simulink model "magnetorquer"  (R2019a)
settings: Solver=ode5  StartTime=0.0  StopTime=10.0  RelTol=1e-3
undefined symbols (not defined in the file or in its folder): sat
libraries: sharedutil x4, simulink x3, vrlib x1
settings Model: Creator=Florian  LastModifiedBy=Florian

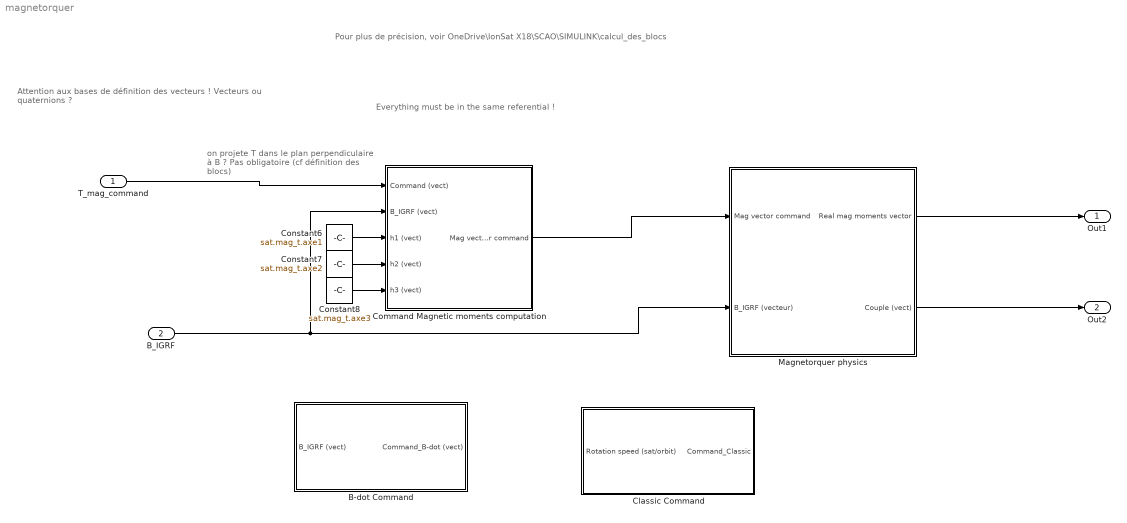
== system magnetorquer ==
  note: Attention aux bases de définition des vecteurs !
      |
      | Vecteurs ou quaternions ?
  note: on projete T dans
      | le plan perpendiculaire à B ?
      | Pas obligatoire (cf définition des blocs)
  note: Everything must be in the same referential !
  note: Pour plus de précision, voir OneDrive\IonSat X18\SCAO\SIMULINK\calcul_des_blocs
  T_mag_command : Inport
  B_IGRF : Inport  Port=2
  B-dot Command : Subsystem
  Classic Command : Subsystem
  Command Magnetic moments computation : Subsystem
  Constant6 : Constant  Value=sat.mag_t.axe1
  Constant7 : Constant  Value=sat.mag_t.axe2
  Constant8 : Constant  Value=sat.mag_t.axe3
  Magnetorquer physics : Subsystem
  Out1 : Outport
  Out2 : Outport  Port=2
  wires:
  Magnetorquer physics/1(Real mag moments vector) -> Out1/1
  Magnetorquer physics/2(Couple (vect)) -> Out2/1
  B_IGRF/1 -> Magnetorquer physics/2(B_IGRF (vecteur)), Command Magnetic moments computation/2(B_IGRF (vect))
  T_mag_command/1 -> Command Magnetic moments computation/1(Command (vect))
  Constant6/1 -> Command Magnetic moments computation/3(h1 (vect))
  Constant7/1 -> Command Magnetic moments computation/4(h2 (vect))
  Constant8/1 -> Command Magnetic moments computation/5(h3 (vect))
  Command Magnetic moments computation/1(Mag vector command) -> Magnetorquer physics/1(Mag vector command)

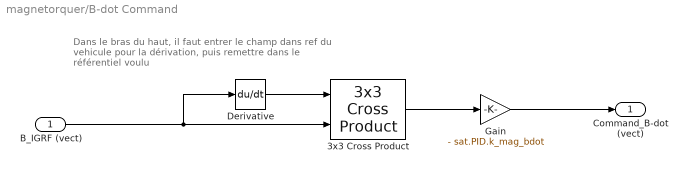
== system magnetorquer/B-dot Command ==
  note: Dans le bras du haut, il faut entrer le champ
      | dans ref du vehicule pour la dérivation, puis remettre
      | dans le référentiel voulu
  B_IGRF (vect) : Inport
  3x3 Cross Product : sharedutil/3x3 Cross Product  aMode=aMode
      settings: SourceProductBaseCode=AE
  Derivative : Derivative
  Gain : Gain  Gain=- sat.PID.k_mag_bdot
  Command_B-dot (vect) : Outport  VectorParamsAs1DForOutWhenUnconnected=off
  wires:
  Derivative/1 -> 3x3 Cross Product/1
  Gain/1 -> Command_B-dot (vect)/1
  B_IGRF (vect)/1 -> Derivative/1, 3x3 Cross Product/2
  3x3 Cross Product/1 -> Gain/1

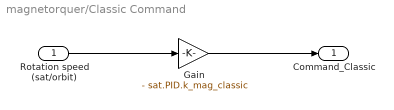
== system magnetorquer/Classic Command ==
  Rotation speed (sat/orbit) : Inport
  Gain : Gain  Gain=- sat.PID.k_mag_classic
  Command_Classic : Outport  VectorParamsAs1DForOutWhenUnconnected=off
  wires:
  Rotation speed (sat/orbit)/1 -> Gain/1
  Gain/1 -> Command_Classic/1

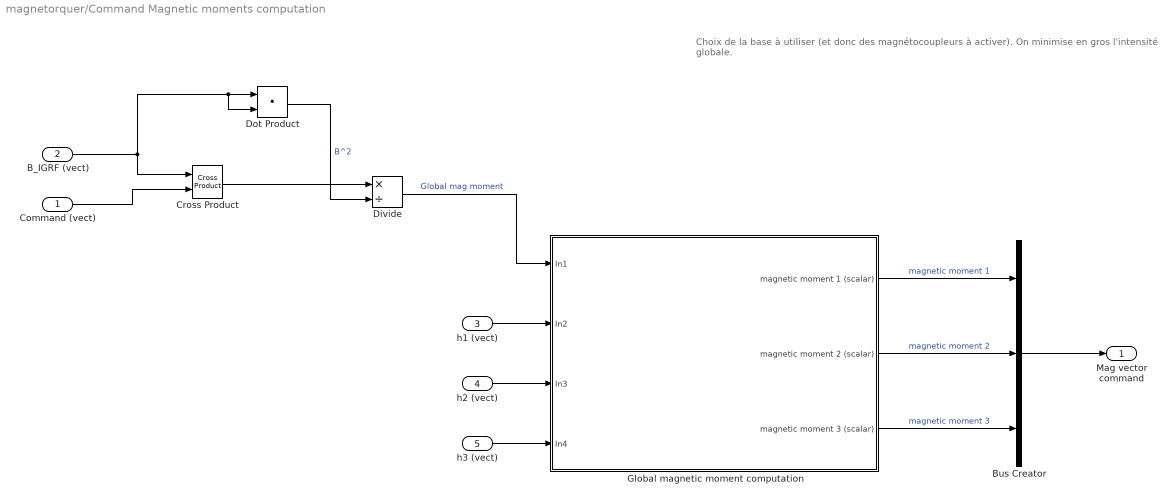
== system magnetorquer/Command Magnetic moments computation ==
  note: Choix de la base à utiliser (et donc des magnétocoupleurs à activer). On minimise en gros l'intensité globale.
  Command (vect) : Inport
  B_IGRF (vect) : Inport  Port=2
  h1 (vect) : Inport  Port=3
  h2 (vect) : Inport  Port=4
  h3 (vect) : Inport  Port=5
  Bus Creator : BusCreator  Inputs=3
  Cross Product : vrlib/Utilities/Cross Product
      settings: SourceProductName=Simulink
  Divide : Product  Inputs=*/
  Dot Product : DotProduct  InputSameDT=on  OutDataTypeStr=Inherit: Inherit via internal rule
  Global magnetic moment computation : Subsystem
  Mag vector command : Outport  VectorParamsAs1DForOutWhenUnconnected=off
  wires:
  B_IGRF (vect)/1 -> Dot Product/2, Dot Product/1, Cross Product/1
  Command (vect)/1 -> Cross Product/2
  Dot Product/1 -> Divide/2  "B^2"
  Cross Product/1 -> Divide/1
  Divide/1 -> Global magnetic moment computation/1(In1)  "Global mag moment"
  h1 (vect)/1 -> Global magnetic moment computation/2(In2)
  h2 (vect)/1 -> Global magnetic moment computation/3(In3)
  h3 (vect)/1 -> Global magnetic moment computation/4(In4)
  Global magnetic moment computation/2(magnetic moment 2 (scalar)) -> Bus Creator/2  "magnetic moment 2"
  Global magnetic moment computation/3(magnetic moment 3 (scalar)) -> Bus Creator/3  "magnetic moment 3"
  Global magnetic moment computation/1(magnetic moment 1 (scalar)) -> Bus Creator/1  "magnetic moment 1"
  Bus Creator/1 -> Mag vector command/1

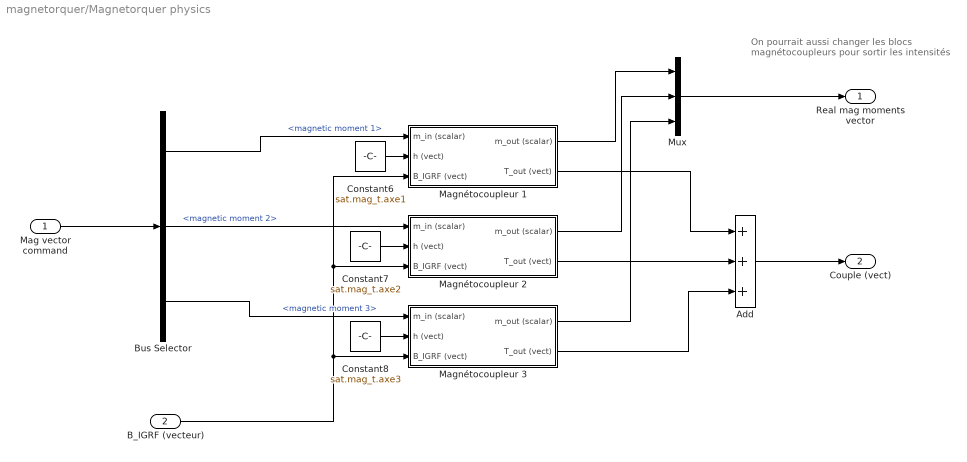
== system magnetorquer/Magnetorquer physics ==
  note: On pourrait aussi changer les blocs
      | magnétocoupleurs pour sortir les intensités
  Mag vector command : Inport
  B_IGRF (vecteur) : Inport  Port=2
  Add : Sum  Inputs=+++
  Bus Selector : BusSelector  OutputSignals=magnetic moment 1,magnetic moment 2,magnetic moment 3
  Constant6 : Constant  Value=sat.mag_t.axe1
  Constant7 : Constant  Value=sat.mag_t.axe2
  Constant8 : Constant  Value=sat.mag_t.axe3
  Magnétocoupleur 1 : Subsystem
  Magnétocoupleur 2 : Subsystem
  Magnétocoupleur 3 : Subsystem
  Mux : Mux  Inputs=3
  Real mag moments vector : Outport  VectorParamsAs1DForOutWhenUnconnected=off
  Couple (vect) : Outport  Port=2  VectorParamsAs1DForOutWhenUnconnected=off
  wires:
  Constant6/1 -> Magnétocoupleur 1/2(h (vect))
  B_IGRF (vecteur)/1 -> Magnétocoupleur 1/3(B_IGRF (vect)), Magnétocoupleur 2/3(B_IGRF (vect)), Magnétocoupleur 3/3(B_IGRF (vect))
  Constant7/1 -> Magnétocoupleur 2/2(h (vect))
  Magnétocoupleur 2/1(m_out (scalar)) -> Mux/2
  Add/1 -> Couple (vect)/1
  Magnétocoupleur 1/2(T_out (vect)) -> Add/1
  Magnétocoupleur 2/2(T_out (vect)) -> Add/2
  Magnétocoupleur 3/2(T_out (vect)) -> Add/3
  Mux/1 -> Real mag moments vector/1
  Magnétocoupleur 1/1(m_out (scalar)) -> Mux/1
  Magnétocoupleur 3/1(m_out (scalar)) -> Mux/3
  Constant8/1 -> Magnétocoupleur 3/2(h (vect))
  Mag vector command/1 -> Bus Selector/1
  Bus Selector/1 -> Magnétocoupleur 1/1(m_in (scalar))  "<magnetic moment 1>"
  Bus Selector/2 -> Magnétocoupleur 2/1(m_in (scalar))  "<magnetic moment 2>"
  Bus Selector/3 -> Magnétocoupleur 3/1(m_in (scalar))  "<magnetic moment 3>"

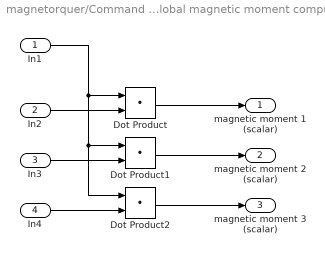
== system magnetorquer/Command Magnetic moments computation/Global magnetic moment computation ==
  In1 : Inport
  In2 : Inport  Port=2
  In3 : Inport  Port=3
  In4 : Inport  Port=4
  Dot Product : DotProduct  InputSameDT=on  OutDataTypeStr=Inherit: Inherit via internal rule
  Dot Product1 : DotProduct  InputSameDT=on  OutDataTypeStr=Inherit: Inherit via internal rule
  Dot Product2 : DotProduct  InputSameDT=on  OutDataTypeStr=Inherit: Inherit via internal rule
  magnetic moment 1 (scalar) : Outport
  magnetic moment 2 (scalar) : Outport  Port=2
  magnetic moment 3 (scalar) : Outport  Port=3
  wires:
  In1/1 -> Dot Product2/1, Dot Product1/1, Dot Product/1
  In2/1 -> Dot Product/2
  In3/1 -> Dot Product1/2
  In4/1 -> Dot Product2/2
  Dot Product/1 -> magnetic moment 1 (scalar)/1
  Dot Product1/1 -> magnetic moment 2 (scalar)/1
  Dot Product2/1 -> magnetic moment 3 (scalar)/1

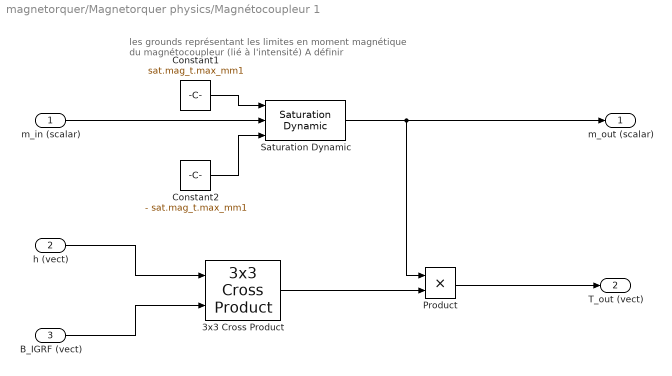
== system magnetorquer/Magnetorquer physics/Magnétocoupleur 1 ==
  note: les grounds représentant les limites en
      |  moment magnétique du magnétocoupleur (lié à l'intensité)
      | A définir
  m_in (scalar) : Inport
  h (vect) : Inport  Port=2
  B_IGRF (vect) : Inport  Port=3
  3x3 Cross Product : sharedutil/3x3 Cross Product  aMode=aMode
      settings: SourceProductBaseCode=AE
  Constant1 : Constant  Value=sat.mag_t.max_mm1
  Constant2 : Constant  Value=- sat.mag_t.max_mm1
  Product : Product
  Saturation Dynamic : simulink/Discontinuities/Saturation Dynamic  OutMin=[]  OutMax=[]  OutDataTypeStr=Inherit: Same as second input  OutDataType=fixdt(1, 16)  OutScaling=2^-10  DoSatur=off
  m_out (scalar) : Outport  VectorParamsAs1DForOutWhenUnconnected=off
  T_out (vect) : Outport  Port=2  VectorParamsAs1DForOutWhenUnconnected=off
  wires:
  h (vect)/1 -> 3x3 Cross Product/1
  B_IGRF (vect)/1 -> 3x3 Cross Product/2
  m_in (scalar)/1 -> Saturation Dynamic/2
  Constant2/1 -> Saturation Dynamic/3
  Constant1/1 -> Saturation Dynamic/1
  Saturation Dynamic/1 -> Product/1, m_out (scalar)/1
  3x3 Cross Product/1 -> Product/2
  Product/1 -> T_out (vect)/1

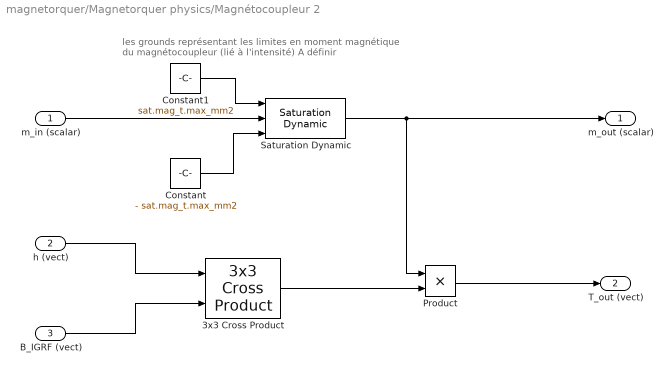
== system magnetorquer/Magnetorquer physics/Magnétocoupleur 2 ==
  note: les grounds représentant les limites en
      |  moment magnétique du magnétocoupleur (lié à l'intensité)
      | A définir
  m_in (scalar) : Inport
  h (vect) : Inport  Port=2
  B_IGRF (vect) : Inport  Port=3
  3x3 Cross Product : sharedutil/3x3 Cross Product  aMode=aMode
      settings: SourceProductBaseCode=AE
  Constant : Constant  Value=- sat.mag_t.max_mm2
  Constant1 : Constant  Value=sat.mag_t.max_mm2
  Product : Product
  Saturation Dynamic : simulink/Discontinuities/Saturation Dynamic  OutMin=[]  OutMax=[]  OutDataTypeStr=Inherit: Same as second input  OutDataType=fixdt(1, 16)  OutScaling=2^-10  DoSatur=off
  m_out (scalar) : Outport  VectorParamsAs1DForOutWhenUnconnected=off
  T_out (vect) : Outport  Port=2  VectorParamsAs1DForOutWhenUnconnected=off
  wires:
  h (vect)/1 -> 3x3 Cross Product/1
  B_IGRF (vect)/1 -> 3x3 Cross Product/2
  m_in (scalar)/1 -> Saturation Dynamic/2
  Constant/1 -> Saturation Dynamic/3
  Constant1/1 -> Saturation Dynamic/1
  Saturation Dynamic/1 -> Product/1, m_out (scalar)/1
  3x3 Cross Product/1 -> Product/2
  Product/1 -> T_out (vect)/1

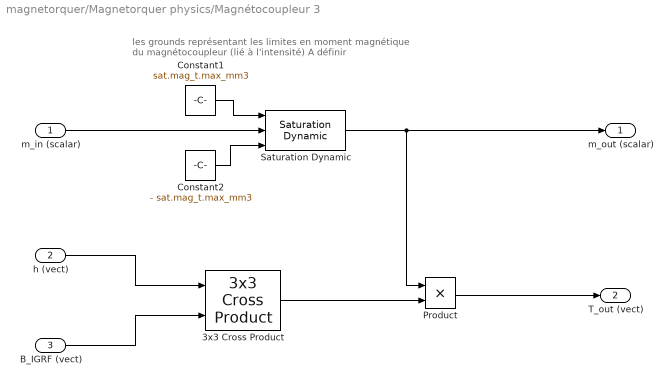
== system magnetorquer/Magnetorquer physics/Magnétocoupleur 3 ==
  note: les grounds représentant les limites en
      |  moment magnétique du magnétocoupleur (lié à l'intensité)
      | A définir
  m_in (scalar) : Inport
  h (vect) : Inport  Port=2
  B_IGRF (vect) : Inport  Port=3
  3x3 Cross Product : sharedutil/3x3 Cross Product  aMode=aMode
      settings: SourceProductBaseCode=AE
  Constant1 : Constant  Value=sat.mag_t.max_mm3
  Constant2 : Constant  Value=- sat.mag_t.max_mm3
  Product : Product
  Saturation Dynamic : simulink/Discontinuities/Saturation Dynamic  OutMin=[]  OutMax=[]  OutDataTypeStr=Inherit: Same as second input  OutDataType=fixdt(1, 16)  OutScaling=2^-10  DoSatur=off
  m_out (scalar) : Outport  VectorParamsAs1DForOutWhenUnconnected=off
  T_out (vect) : Outport  Port=2  VectorParamsAs1DForOutWhenUnconnected=off
  wires:
  h (vect)/1 -> 3x3 Cross Product/1
  B_IGRF (vect)/1 -> 3x3 Cross Product/2
  m_in (scalar)/1 -> Saturation Dynamic/2
  Constant2/1 -> Saturation Dynamic/3
  Constant1/1 -> Saturation Dynamic/1
  Saturation Dynamic/1 -> Product/1, m_out (scalar)/1
  3x3 Cross Product/1 -> Product/2
  Product/1 -> T_out (vect)/1
